simulink model "es2_simulink"  (R2024b)
settings: Solver=VariableStepAuto  StartTime=0.0  StopTime=end_time  RelTol=1e-3
values from neighbouring files (symbols this model uses):
  A = [0 1/Cap; -1/L -R/L]    [init_es2.m]
  B = [0;1/L]    [init_es2.m]
  C = [1 0]    [init_es2.m]
  D = [0]    [init_es2.m]
  L = 10e-3    (= 0.01)    [init_es2.m]
  om = 1*10^3    (= 1000)    [init_es2.m]
  R = 1e3    (= 1000)    [init_es2.m]
  U = 10    [init_es2.m]
  x0 = [x1_0 x2_0]    [init_es2.m]
  x1_0 = 0    [init_es2.m]
undefined symbols (not defined in the file or in its folder): den, num
settings Model: Creator=jacoposini  LastModifiedBy=jacoposini

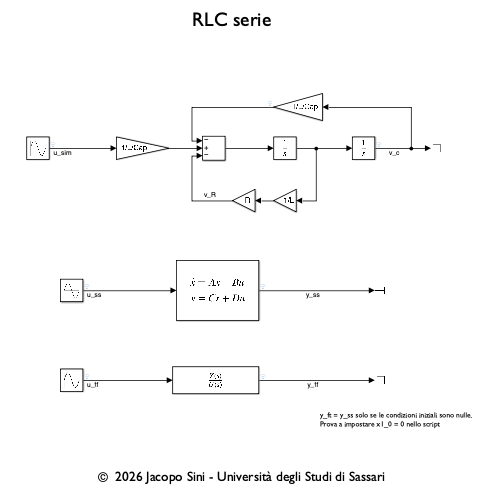
[thumbnail: Simulink's stored preview of the top-level diagram]
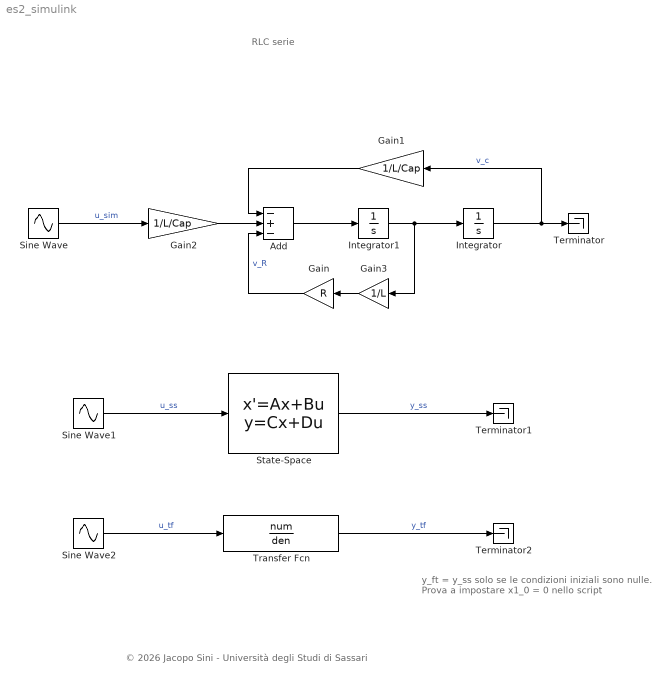
== system es2_simulink ==
  note: y_ft = y_ss solo se le condizioni iniziali sono nulle.
      | Prova a impostare x1_0 = 0 nello script
  note: RLC serie
  note: © 2026 Jacopo Sini - Università degli Studi di Sassari
  Add : Sum  Inputs=-+-
  Gain : Gain  Gain=R
  Gain1 : Gain  Gain=1/L/Cap
  Gain2 : Gain  Gain=1/L/Cap
  Gain3 : Gain  Gain=1/L
  Integrator : Integrator  InitialCondition=x1_0
  Integrator1 : Integrator
  Sine Wave : Sin  Amplitude=U  Frequency=om  SampleTime=0
  Sine Wave1 : Sin  Amplitude=U  Frequency=om  SampleTime=0
  Sine Wave2 : Sin  Amplitude=U  Frequency=om  SampleTime=0
  State-Space : StateSpace  A=A  B=B  C=C  D=D  InitialCondition=x0
  Terminator : Terminator
  Terminator1 : Terminator
  Terminator2 : Terminator
  Transfer Fcn : TransferFcn  Numerator=num  Denominator=den
  wires:
  Integrator/1 -> Gain1/1, Terminator/1  "v_c"
  Sine Wave/1 -> Gain2/1  "u_sim"
  Sine Wave1/1 -> State-Space/1  "u_ss"
  State-Space/1 -> Terminator1/1  "y_ss"
  Gain2/1 -> Add/2
  Gain/1 -> Add/3  "v_R"
  Gain1/1 -> Add/1
  Integrator1/1 -> Gain3/1, Integrator/1
  Sine Wave2/1 -> Transfer Fcn/1  "u_tf"
  Transfer Fcn/1 -> Terminator2/1  "y_tf"
  Add/1 -> Integrator1/1
  Gain3/1 -> Gain/1
